simulink model "YawPathControl"  (R2022b)
settings: Solver=VariableStepAuto  StartTime=0.0  StopTime=10  RelTol=1e-3
undefined symbols (not defined in the file): a11, a12, a21, a22, b11, b12, b21, b22, Cf, Cr, Cs, e2, Gn, J, Lf, Lr, m, mu, Q, Vref
libraries: cstblocks x4, slpidlib x1
settings Model: Creator=Santo  LastModifiedBy=brianlesko
settings SolverCC: AlgebraicLoopSolver=TrustRegion
settings DataIOCC: ReturnWorkspaceOutputs=off
settings DebuggingCC: UnconnectedInputMsg=warning  UnconnectedOutputMsg=warning  UnconnectedLineMsg=warning  SFMachineParentedDataDiag=warning  ArithmeticOperatorsInVariantConditions=warning
settings ModelReferenceCC: EnableRefExpFcnMdlSchedulingChecks=on
settings SFSimCC: SimUseLocalCustomCode=off  CustomCodeUndefinedFunction=UseInterfaceOnly
settings RTWCC: RTWUseLocalCustomCode=off

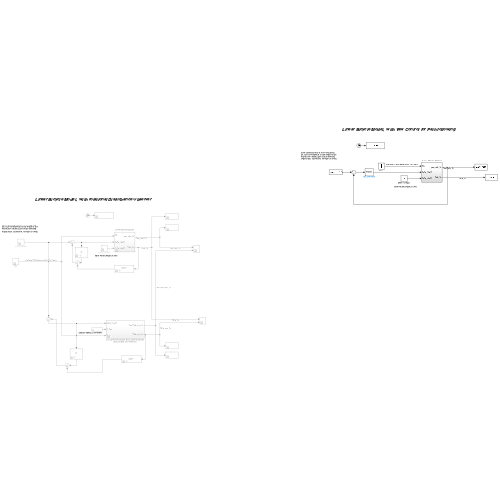
[thumbnail: Simulink's stored preview of the top-level diagram]
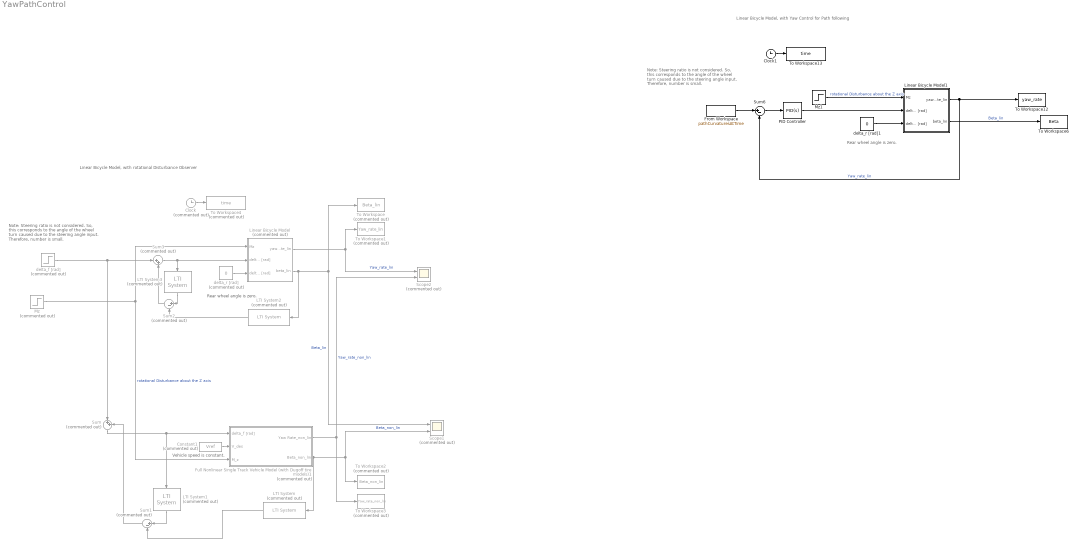
== system YawPathControl ==
  note: Linear Bicycle Model, with rotational Disturbance Observer
  note: Rear wheel angle is zero.
  note: Vehicle speed is constant.
  note: Note: Steering ratio is not considered. So, this corresponds to the angle of the wheel turn caused due to the steering angle input. Therefore, number is small.
  note: Linear Bicycle Model, with Yaw Control for Path following
  note: Rear wheel angle is zero.
  note: Note: Steering ratio is not considered. So, this corresponds to the angle of the wheel turn caused due to the steering angle input. Therefore, number is small.
  Clock : Clock  Commented=on
  Clock1 : Clock
  Constant1 : Constant  Commented=on  Value=Vref
  From Workspace : FromWorkspace  VariableName=pathCurvaturesAtTime
  Full Nonlinear Single Track Vehicle Model (with Dugoff tire models)1 : Subsystem  Commented=on
  LTI System : cstblocks/LTI System  Commented=on  sys=Q/Gn  IC=[]
  LTI System1 : cstblocks/LTI System  Commented=on  sys=Q  IC=[]
  LTI System2 : cstblocks/LTI System  Commented=on  sys=Q/Gn  IC=[]
  LTI System3 : cstblocks/LTI System  Commented=on  sys=Q  IC=[]
  Linear Bicycle Model : Subsystem  Commented=on
  Linear Bicycle Model1 : Subsystem
  Mz : Step  Commented=on  Time=5  After=100  SampleTime=0
  Mz1 : Step  Time=5  After=100  SampleTime=0
  PID Controller : slpidlib/PID Controller  Controller=PID  Form=Parallel  TimeDomain=Continuous-time  UseExternalTs=off  SampleTime=-1  IntegratorMethod=Forward Euler  FilterMethod=Forward Euler  ControllerParametersSource=internal  P=1.20253324681122  I=42.4205335808931  UseKiTs=off  D=0.00143593410548543  N=287.769955007981  UseFilter=on  TunerSelectOption=Transfer Function Based (PID Tuner App)  InitialConditionSource=internal  InitialConditionForIntegrator=0  InitialConditionForFilter=0  DifferentiatorICPrevScaledInput=0  ExternalReset=none  TrackingMode=off  Kt=1  LimitOutput=off  SatLimitsSource=internal  UpperSaturationLimit=inf  LowerSaturationLimit=-inf  LinearizeAsGain=on  AntiWindupMode=none  Kb=1  LimitIntegrator=off  UpperIntegratorSaturationLimit=inf  LowerIntegratorSaturationLimit=-inf  POutMin=[]  POutMax=[]  IOutMin=[]  IOutMax=[]  DOutMin=[]  DOutMax=[]  NOutMin=[]  NOutMax=[]  SumOutMin=[]  SumOutMax=[]  SaturationOutMin=[]  SaturationOutMax=[]  PParamMin=[]  PParamMax=[]  IParamMin=[]  IParamMax=[]  DParamMin=[]  DParamMax=[]  NParamMin=[]  NParamMax=[]  KbParamMin=[]  KbParamMax=[]  KtParamMin=[]  KtParamMax=[]  KbOutMin=[]  KbOutMax=[]  KtOutMin=[]  KtOutMax=[]  IntegratorOutMin=[]  IntegratorOutMax=[]  FilterOutMin=[]  FilterOutMax=[]  SumI1OutMin=[]  SumI1OutMax=[]  SumI2OutMin=[]  SumI2OutMax=[]  SumI3OutMin=[]  SumI3OutMax=[]  SumI4OutMin=[]  SumI4OutMax=[]  SumDOutMin=[]  SumDOutMax=[]  DifferentiatorOutMin=[]  DifferentiatorOutMax=[]  FilterDiffOutCoefMin=[]  FilterDiffOutCoefMax=[]  ReciprocalOutMin=[]  ReciprocalOutMax=[]  SumDenOutMin=[]  SumDenOutMax=[]  SumNumOutMin=[]  SumNumOutMax=[]  DivideOutMin=[]  DivideOutMax=[]  UdiffTsProdOutMin=[]  UdiffTsProdOutMax=[]  NTsProdOutMin=[]  NTsProdOutMax=[]  UintegralTsProdOutMin=[]  UintegralTsProdOutMax=[]  UngainTsProdOutMin=[]  UngainTsProdOutMax=[]  ClampingZeroOutDataTypeStr=Inherit: Inherit via back propagation  ClampingZeroOutMin=[]  ClampingZeroOutMax=[]  FilterDenConstantOutDataTypeStr=Inherit: Inherit via back propagation  FilterDenConstantOutMin=[]  FilterDenConstantOutMax=[]  PCopyOutDataTypeStr=Inherit: Inherit via back propagation  PCopyOutMin=[]  PCopyOutMax=[]  NCopyOutDataTypeStr=Inherit: Inherit via back propagation  NCopyOutMin=[]  NCopyOutMax=[]  IntegratorContinuousStateAttributes=''  IntegratorStateMustResolveToSignalObject=off  IntegratorRTWStateStorageClass=Auto  FilterContinuousStateAttributes=''  FilterStateMustResolveToSignalObject=off  FilterRTWStateStorageClass=Auto  ParallelPVariant=InternalParameters  IdealPVariant=Disabled  IVariant=InternalParameters  DVariant=InternalParameters  IntegratorVariant=Continuous  SatVariant=Disabled  AWVariant=Passthrough  PCopyVariant=Disabled  TRVariant=Disabled  FdbkBlocksVariant=Forward  IdealPFdbkVariant=Disabled  SatFdbkVariant=Disabled  DerivativeFilterVariant=ContFilter  NVariant=InternalParameters  NCopyVariant=Disabled  FilterICVariant=InternalICsFilter  IntegratorICVariant=InternalICs  ExternalResetVariant=Disabled  TRSumVariant=Passthrough  SumFdbkVariant=Disabled  SumVariant=Sum_PID  TsampFilterVariant=InternalTs  TsampNgainVariant=Passthrough  TsampIntegralVariant=Passthrough  ExternalSaturationOutDataTypeStr=Inherit: Same as second input
  Scope1 : Scope  Commented=on  NumInputPorts=2
  Scope2 : Scope  Commented=on  NumInputPorts=2
  Sum : Sum  Commented=on  Inputs=|++
  Sum1 : Sum  Commented=on  Inputs=|+-
  Sum2 : Sum  Commented=on  Inputs=|+-
  Sum3 : Sum  Commented=on  Inputs=|++
  Sum6 : Sum  Inputs=|+-
  To Workspace : ToWorkspace  Commented=on  VariableName=Beta_lin  SampleTime=-1
  To Workspace1 : ToWorkspace  Commented=on  VariableName=Yaw_rate_lin  SampleTime=-1
  To Workspace12 : ToWorkspace  VariableName=yaw_rate  SampleTime=-1
  To Workspace13 : ToWorkspace  VariableName=time  SampleTime=-1
  To Workspace2 : ToWorkspace  Commented=on  VariableName=Beta_non_lin  SampleTime=-1
  To Workspace3 : ToWorkspace  Commented=on  VariableName=Yaw_rate_non_lin  SampleTime=-1
  To Workspace4 : ToWorkspace  Commented=on  VariableName=time  SampleTime=-1
  To Workspace6 : ToWorkspace  VariableName=Beta  SampleTime=-1
  delta_f [rad] : Step  Commented=on  After=5*pi/180  SampleTime=0
  delta_r [rad] : Constant  Commented=on  Value=0
  delta_r [rad]1 : Constant  Value=0
  wires:
  delta_r [rad]/1 -> Linear Bicycle Model/3(delta_r [rad])
  Linear Bicycle Model/1(yaw_rate_lin) -> To Workspace1/1, Scope2/1  "Yaw_rate_lin"
  Linear Bicycle Model/2(beta_lin) -> LTI System2/1, To Workspace/1, Scope1/1  "Beta_lin"
  delta_f [rad]/1 -> Sum3/1, Sum/1
  Full Nonlinear Single Track Vehicle Model (with Dugoff tire models)1/1(Yaw Rate_non_lin) -> To Workspace3/1, Scope2/2  "Yaw_rate_non_lin"
  Mz/1 -> Full Nonlinear Single Track Vehicle Model (with Dugoff tire models)1/3(M_z), Linear Bicycle Model/1(Mz)  "rotational Disturbance about the Z axis"
  Constant1/1 -> Full Nonlinear Single Track Vehicle Model (with Dugoff tire models)1/2("V_des ")
  Full Nonlinear Single Track Vehicle Model (with Dugoff tire models)1/2(Beta_non_lin) -> LTI System/1, To Workspace2/1, Scope1/2  "Beta_non_lin"
  Clock/1 -> To Workspace4/1
  Sum/1 -> Full Nonlinear Single Track Vehicle Model (with Dugoff tire models)1/1(delta_f [rad]), LTI System1/1
  Sum1/1 -> Sum/2
  LTI System1/1 -> Sum1/1
  LTI System/1 -> Sum1/2
  LTI System3/1 -> Sum2/1
  LTI System2/1 -> Sum2/2
  Sum3/1 -> Linear Bicycle Model/2(delta_f [rad]), LTI System3/1
  Sum2/1 -> Sum3/2
  Linear Bicycle Model1/2(beta_lin) -> To Workspace6/1  "Beta_lin"
  Linear Bicycle Model1/1(yaw_rate_lin) -> To Workspace12/1, Sum6/2  "Yaw_rate_lin"
  Mz1/1 -> Linear Bicycle Model1/1(Mz)  "rotational Disturbance about the Z axis"
  Clock1/1 -> To Workspace13/1
  Sum6/1 -> PID Controller/1
  delta_r [rad]1/1 -> Linear Bicycle Model1/3(delta_r [rad])
  PID Controller/1 -> Linear Bicycle Model1/2(delta_f [rad])
  From Workspace/1 -> Sum6/1

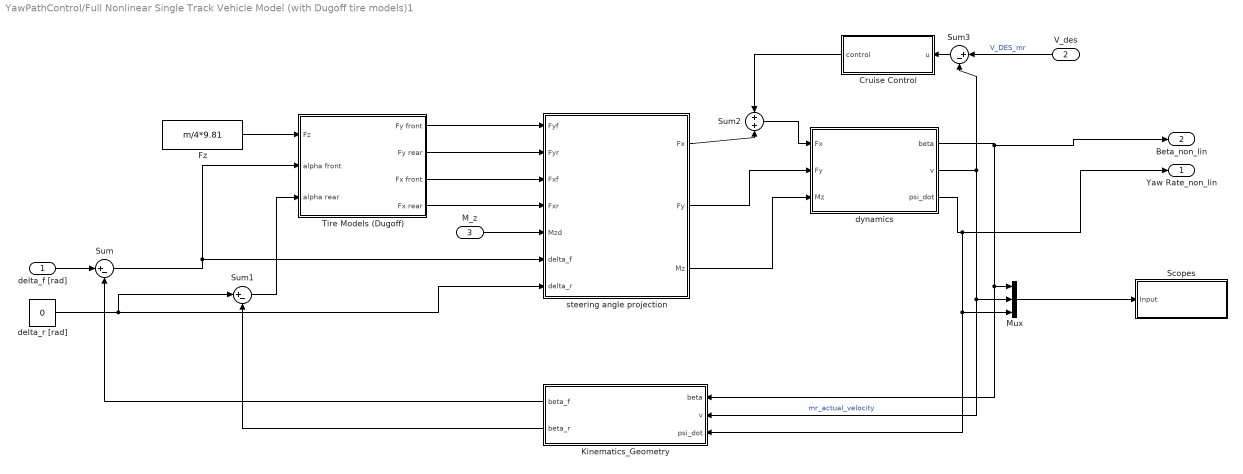
== system YawPathControl/Full Nonlinear Single Track Vehicle Model (with Dugoff tire models)1 ==
  delta_f [rad] : Inport
  "V_des " : Inport  Port=2
  M_z : Inport  Port=3
  Cruise Control : Subsystem
  Fz : Constant  Value=m/4*9.81
  Kinematics_Geometry : Subsystem
  Mux : Mux  Inputs=3
  Scopes : Subsystem
  Sum : Sum  Inputs=|+-  SaturateOnIntegerOverflow=on
  Sum1 : Sum  Inputs=|+-  SaturateOnIntegerOverflow=on
  Sum2 : Sum
  Sum3 : Sum  Inputs=|+-  SaturateOnIntegerOverflow=on
  Tire Models (Dugoff) : Subsystem
  delta_r [rad] : Constant  Value=0
  dynamics : Subsystem
  steering angle projection : Subsystem
  Yaw Rate_non_lin : Outport  VectorParamsAs1DForOutWhenUnconnected=off
  Beta_non_lin : Outport  Port=2  VectorParamsAs1DForOutWhenUnconnected=off
  wires:
  Sum3/1 -> Cruise Control/1(u)
  "V_des "/1 -> Sum3/1  "V_DES_mr"
  steering angle projection/1(Fx) -> Sum2/2
  steering angle projection/2(Fy) -> dynamics/2(Fy)
  steering angle projection/3(Mz) -> dynamics/3(Mz)
  dynamics/2(v) -> Mux/2, Kinematics_Geometry/2(v), Sum3/2  "mr_actual_velocity"
  dynamics/3(psi_dot) -> Yaw Rate_non_lin/1, Mux/3, Kinematics_Geometry/3(psi_dot)
  delta_f [rad]/1 -> Sum/1
  delta_r [rad]/1 -> Sum1/1, steering angle projection/7(delta_r)
  Sum1/1 -> Tire Models (Dugoff)/3(alpha rear)
  Sum/1 -> Tire Models (Dugoff)/2(alpha front), steering angle projection/6(delta_f)
  Mux/1 -> Scopes/1(Input)
  Kinematics_Geometry/1(beta_f) -> Sum/2
  Kinematics_Geometry/2(beta_r) -> Sum1/2
  Fz/1 -> Tire Models (Dugoff)/1(Fz)
  Tire Models (Dugoff)/1(Fy front) -> steering angle projection/1(Fyf)
  Tire Models (Dugoff)/2(Fy rear) -> steering angle projection/2(Fyr)
  Tire Models (Dugoff)/3(Fx front) -> steering angle projection/3(Fxf)
  Tire Models (Dugoff)/4(Fx rear) -> steering angle projection/4(Fxr)
  M_z/1 -> steering angle projection/5(Mzd)
  Cruise Control/1(control) -> Sum2/1
  Sum2/1 -> dynamics/1(Fx)
  dynamics/1(beta) -> Beta_non_lin/1, Kinematics_Geometry/1(beta), Mux/1

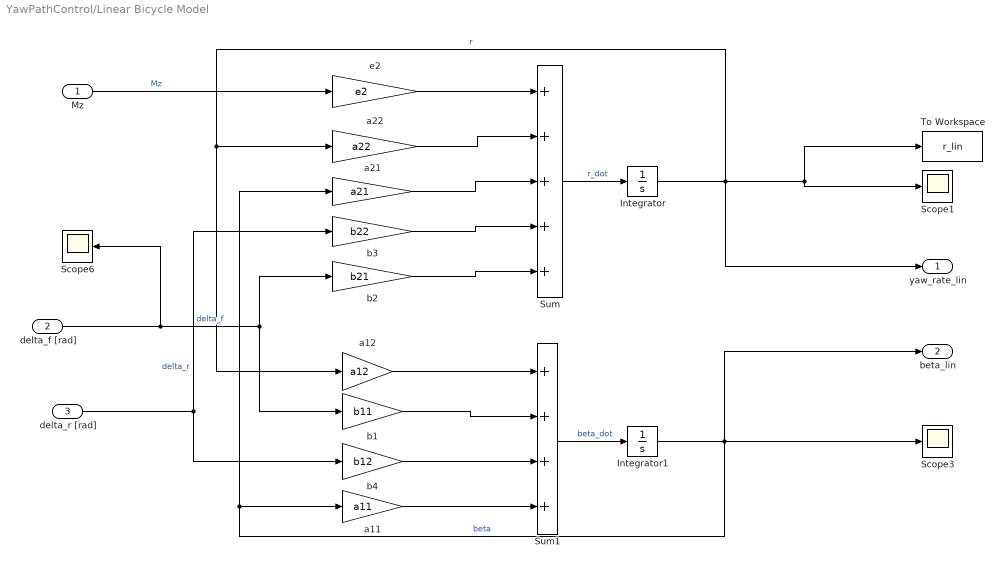
== system YawPathControl/Linear Bicycle Model ==
  Mz : Inport
  delta_f [rad] : Inport  Port=2
  delta_r [rad] : Inport  Port=3
  Integrator : Integrator
  Integrator1 : Integrator
  Scope1 : Scope
  Scope3 : Scope
  Scope6 : Scope
  Sum : Sum  Inputs=+++++
  Sum1 : Sum  Inputs=++++
  To Workspace : ToWorkspace  VariableName=r_lin  SaveFormat=Timeseries  SampleTime=-1
  a11 : Gain  Gain=a11
  a12 : Gain  Gain=a12
  a21 : Gain  Gain=a21
  a22 : Gain  Gain=a22
  b1 : Gain  Gain=b11
  b2 : Gain  Gain=b21
  b3 : Gain  Gain=b22
  b4 : Gain  Gain=b12
  e2 : Gain  Gain=e2
  yaw_rate_lin : Outport  VectorParamsAs1DForOutWhenUnconnected=off
  beta_lin : Outport  Port=2  VectorParamsAs1DForOutWhenUnconnected=off
  wires:
  Sum1/1 -> Integrator1/1  "beta_dot"
  Sum/1 -> Integrator/1  "r_dot"
  a21/1 -> Sum/3
  a11/1 -> Sum1/4
  a12/1 -> Sum1/1
  a22/1 -> Sum/2
  b1/1 -> Sum1/2
  b2/1 -> Sum/5
  delta_f [rad]/1 -> b1/1, b2/1, Scope6/1  "delta_f"
  Integrator1/1 -> beta_lin/1, Scope3/1, a11/1, a21/1  "beta"
  Integrator/1 -> yaw_rate_lin/1, Scope1/1, To Workspace/1, a22/1, a12/1  "r"
  delta_r [rad]/1 -> b3/1, b4/1  "delta_r"
  b3/1 -> Sum/4
  b4/1 -> Sum1/3
  Mz/1 -> e2/1  "Mz"
  e2/1 -> Sum/1

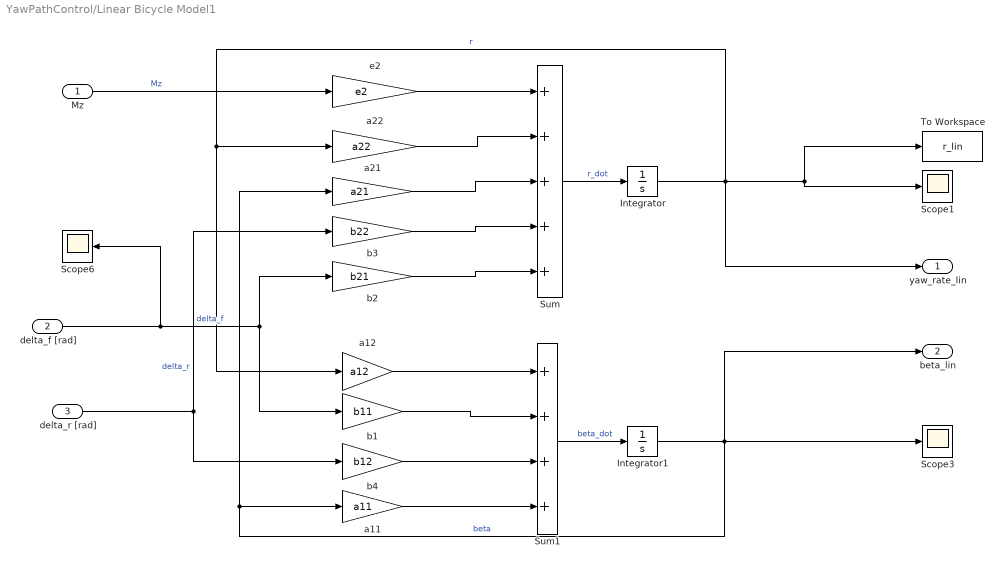
== system YawPathControl/Linear Bicycle Model1 ==
  Mz : Inport
  delta_f [rad] : Inport  Port=2
  delta_r [rad] : Inport  Port=3
  Integrator : Integrator
  Integrator1 : Integrator
  Scope1 : Scope
  Scope3 : Scope
  Scope6 : Scope
  Sum : Sum  Inputs=+++++
  Sum1 : Sum  Inputs=++++
  To Workspace : ToWorkspace  VariableName=r_lin  SaveFormat=Timeseries  SampleTime=-1
  a11 : Gain  Gain=a11
  a12 : Gain  Gain=a12
  a21 : Gain  Gain=a21
  a22 : Gain  Gain=a22
  b1 : Gain  Gain=b11
  b2 : Gain  Gain=b21
  b3 : Gain  Gain=b22
  b4 : Gain  Gain=b12
  e2 : Gain  Gain=e2
  yaw_rate_lin : Outport  VectorParamsAs1DForOutWhenUnconnected=off
  beta_lin : Outport  Port=2  VectorParamsAs1DForOutWhenUnconnected=off
  wires:
  Sum1/1 -> Integrator1/1  "beta_dot"
  Sum/1 -> Integrator/1  "r_dot"
  a21/1 -> Sum/3
  a11/1 -> Sum1/4
  a12/1 -> Sum1/1
  a22/1 -> Sum/2
  b1/1 -> Sum1/2
  b2/1 -> Sum/5
  delta_f [rad]/1 -> b1/1, b2/1, Scope6/1  "delta_f"
  Integrator1/1 -> beta_lin/1, Scope3/1, a11/1, a21/1  "beta"
  Integrator/1 -> yaw_rate_lin/1, Scope1/1, To Workspace/1, a22/1, a12/1  "r"
  delta_r [rad]/1 -> b3/1, b4/1  "delta_r"
  b3/1 -> Sum/4
  b4/1 -> Sum1/3
  Mz/1 -> e2/1  "Mz"
  e2/1 -> Sum/1

== system YawPathControl/Full Nonlinear Single Track Vehicle Model (with Dugoff tire models)1/Cruise Control ==
  u : Inport
  Gain : Gain  Gain=40000  SaturateOnIntegerOverflow=on  OutDataTypeStr=Inherit: Same as input  ParamDataTypeStr=Inherit: Same as input
  Gain1 : Gain  Gain=4000  SaturateOnIntegerOverflow=on  OutDataTypeStr=Inherit: Same as input  ParamDataTypeStr=Inherit: Same as input
  Integrator : Integrator
  Sum : Sum  SaturateOnIntegerOverflow=on
  control : Outport  VectorParamsAs1DForOutWhenUnconnected=off
  wires:
  u/1 -> Gain/1, Integrator/1
  Integrator/1 -> Gain1/1
  Gain1/1 -> Sum/2
  Gain/1 -> Sum/1
  Sum/1 -> control/1

== system YawPathControl/Full Nonlinear Single Track Vehicle Model (with Dugoff tire models)1/Kinematics_Geometry ==
  beta : Inport
  v : Inport  Port=2
  psi_dot : Inport  Port=3
  Mux : Mux  Inputs=3
  beta_f Calc : Fcn  Expr=atan( tan(u(1)) + u(3)*Lf/(u(2)*cos(u(1))) )
  beta_r Calc : Fcn  Expr=atan( tan(u(1)) - u(3)*Lr/(u(2)*cos(u(1))) )
  beta_f : Outport  VectorParamsAs1DForOutWhenUnconnected=off
  beta_r : Outport  Port=2  VectorParamsAs1DForOutWhenUnconnected=off
  wires:
  beta/1 -> Mux/1
  v/1 -> Mux/2
  psi_dot/1 -> Mux/3
  Mux/1 -> beta_f Calc/1, beta_r Calc/1
  beta_r Calc/1 -> beta_r/1
  beta_f Calc/1 -> beta_f/1

== system YawPathControl/Full Nonlinear Single Track Vehicle Model (with Dugoff tire models)1/Scopes ==
  Input : Inport
  Demux : Demux  Outputs=3
      settings: DisplayOption=none
  Distance Traveled : Subsystem
  beta : Scope
  speed : Scope
  yaw Calc : Integrator
  yaw angle : Scope
  yaw rate : Scope
  wires:
  Input/1 -> Demux/1
  Demux/1 -> beta/1, Distance Traveled/2(beta)
  Demux/2 -> speed/1, Distance Traveled/1(V)
  Demux/3 -> yaw rate/1, yaw Calc/1
  yaw Calc/1 -> yaw angle/1, Distance Traveled/3(psi)

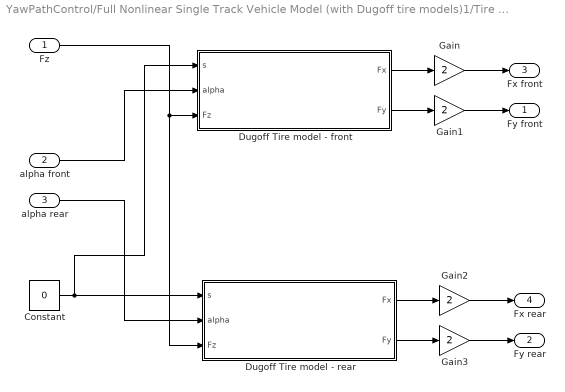
== system YawPathControl/Full Nonlinear Single Track Vehicle Model (with Dugoff tire models)1/Tire Models (Dugoff) ==
  Fz : Inport
  alpha front : Inport  Port=2
  alpha rear : Inport  Port=3
  Constant : Constant  Value=0
  Dugoff Tire model - front : Subsystem
  Dugoff Tire model - rear : Subsystem
  Gain{,1..3} (4 alike) : Gain  Gain=2
  Fy front : Outport  VectorParamsAs1DForOutWhenUnconnected=off
  Fy rear : Outport  Port=2  VectorParamsAs1DForOutWhenUnconnected=off
  Fx front : Outport  Port=3  VectorParamsAs1DForOutWhenUnconnected=off
  Fx rear : Outport  Port=4  VectorParamsAs1DForOutWhenUnconnected=off
  wires:
  alpha rear/1 -> Dugoff Tire model - rear/2(alpha)
  alpha front/1 -> Dugoff Tire model - front/2(alpha)
  Fz/1 -> Dugoff Tire model - front/3(Fz), Dugoff Tire model - rear/3(Fz)
  Constant/1 -> Dugoff Tire model - front/1(s), Dugoff Tire model - rear/1(s)
  Dugoff Tire model - rear/2(Fy) -> Gain3/1
  Dugoff Tire model - rear/1(Fx) -> Gain2/1
  Dugoff Tire model - front/2(Fy) -> Gain1/1
  Dugoff Tire model - front/1(Fx) -> Gain/1
  Gain/1 -> Fx front/1
  Gain1/1 -> Fy front/1
  Gain2/1 -> Fx rear/1
  Gain3/1 -> Fy rear/1

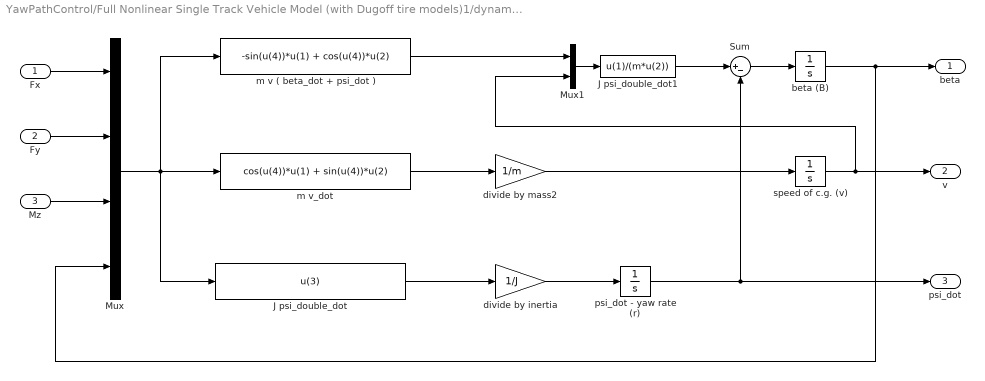
== system YawPathControl/Full Nonlinear Single Track Vehicle Model (with Dugoff tire models)1/dynamics ==
  Fx : Inport
  Fy : Inport  Port=2
  Mz : Inport  Port=3
  J psi_double_dot : Fcn  Expr=u(3)
  J psi_double_dot1 : Fcn  Expr=u(1)/(m*u(2))
  Mux : Mux
  Mux1 : Mux  Inputs=2
  Sum : Sum  Inputs=|+-  SaturateOnIntegerOverflow=on
  beta (B) : Integrator
  divide by inertia : Gain  Gain=1/J  SaturateOnIntegerOverflow=on  OutDataTypeStr=Inherit: Same as input  ParamDataTypeStr=Inherit: Same as input
  divide by mass2 : Gain  Gain=1/m  SaturateOnIntegerOverflow=on  OutDataTypeStr=Inherit: Same as input  ParamDataTypeStr=Inherit: Same as input
  m v ( beta_dot + psi_dot ) : Fcn  Expr=-sin(u(4))*u(1) + cos(u(4))*u(2)
  m v_dot : Fcn  Expr=cos(u(4))*u(1) + sin(u(4))*u(2)
  psi_dot - yaw rate (r) : Integrator
  speed of c.g. (v) : Integrator  InitialCondition=Vref
  beta : Outport  VectorParamsAs1DForOutWhenUnconnected=off
  v : Outport  Port=2  VectorParamsAs1DForOutWhenUnconnected=off
  psi_dot : Outport  Port=3  VectorParamsAs1DForOutWhenUnconnected=off
  wires:
  Fx/1 -> Mux/1
  Fy/1 -> Mux/2
  Mz/1 -> Mux/3
  Mux/1 -> m v ( beta_dot + psi_dot )/1, m v_dot/1, J psi_double_dot/1
  divide by inertia/1 -> psi_dot - yaw rate (r)/1
  Sum/1 -> beta (B)/1
  psi_dot - yaw rate (r)/1 -> Sum/2, psi_dot/1
  divide by mass2/1 -> speed of c.g. (v)/1
  speed of c.g. (v)/1 -> v/1, Mux1/2
  beta (B)/1 -> beta/1, Mux/4
  m v ( beta_dot + psi_dot )/1 -> Mux1/1
  m v_dot/1 -> divide by mass2/1
  J psi_double_dot/1 -> divide by inertia/1
  Mux1/1 -> J psi_double_dot1/1
  J psi_double_dot1/1 -> Sum/1

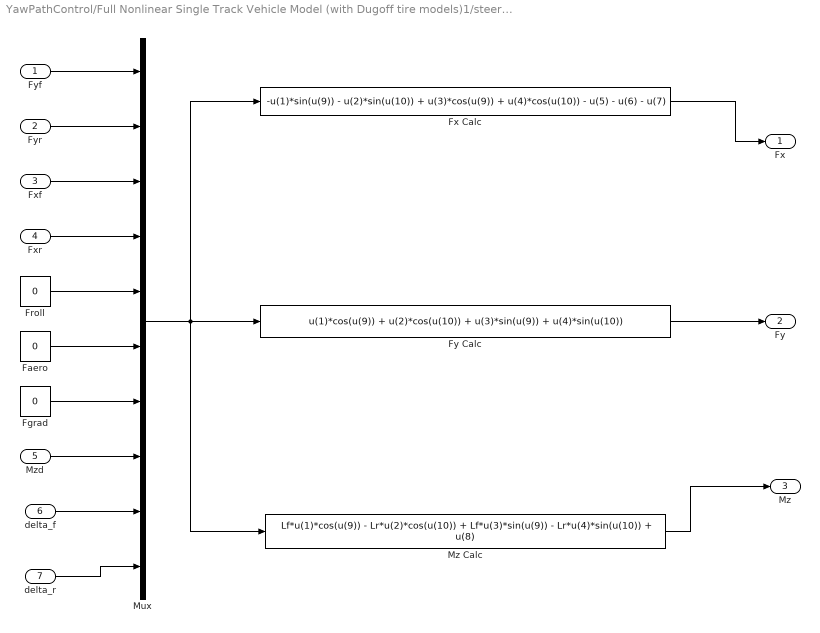
== system YawPathControl/Full Nonlinear Single Track Vehicle Model (with Dugoff tire models)1/steering angle projection ==
  Fyf : Inport
  Fyr : Inport  Port=2
  Fxf : Inport  Port=3
  Fxr : Inport  Port=4
  Mzd : Inport  Port=5
  delta_f : Inport  Port=6
  delta_r : Inport  Port=7
  Faero : Constant  Value=0
  Fgrad : Constant  Value=0
  Froll : Constant  Value=0
  Fx Calc : Fcn  Expr=-u(1)*sin(u(9)) - u(2)*sin(u(10)) + u(3)*cos(u(9)) + u(4)*cos(u(10)) - u(5) - u(6) - u(7)
  Fy Calc : Fcn  Expr=u(1)*cos(u(9)) + u(2)*cos(u(10)) + u(3)*sin(u(9)) + u(4)*sin(u(10))
  Mux : Mux  Inputs=10
  Mz Calc : Fcn  Expr=Lf*u(1)*cos(u(9)) - Lr*u(2)*cos(u(10)) + Lf*u(3)*sin(u(9)) - Lr*u(4)*sin(u(10)) + u(8)
  Fx : Outport  VectorParamsAs1DForOutWhenUnconnected=off
  Fy : Outport  Port=2  VectorParamsAs1DForOutWhenUnconnected=off
  Mz : Outport  Port=3  VectorParamsAs1DForOutWhenUnconnected=off
  wires:
  Fyf/1 -> Mux/1
  Fyr/1 -> Mux/2
  Fxf/1 -> Mux/3
  Fxr/1 -> Mux/4
  Froll/1 -> Mux/5
  Faero/1 -> Mux/6
  Fgrad/1 -> Mux/7
  Mzd/1 -> Mux/8
  delta_f/1 -> Mux/9
  delta_r/1 -> Mux/10
  Fx Calc/1 -> Fx/1
  Mux/1 -> Fx Calc/1, Fy Calc/1, Mz Calc/1
  Fy Calc/1 -> Fy/1
  Mz Calc/1 -> Mz/1

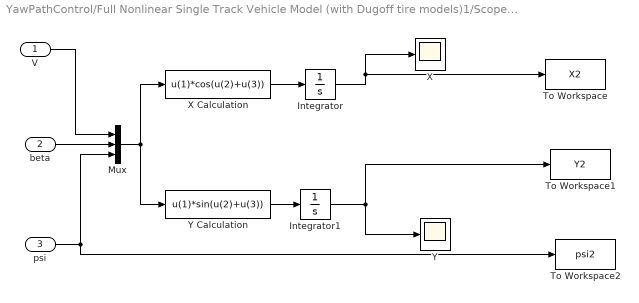
== system YawPathControl/Full Nonlinear Single Track Vehicle Model (with Dugoff tire models)1/Scopes/Distance Traveled ==
  V : Inport
  beta : Inport  Port=2
  psi : Inport  Port=3
  Integrator : Integrator
  Integrator1 : Integrator
  Mux : Mux  Inputs=3
  To Workspace : ToWorkspace  VariableName=X2  SampleTime=-1
  To Workspace1 : ToWorkspace  VariableName=Y2  SampleTime=-1
  To Workspace2 : ToWorkspace  VariableName=psi2  SampleTime=-1
  X : Scope
  X Calculation : Fcn  Expr=u(1)*cos(u(2)+u(3))
  Y : Scope
  Y Calculation : Fcn  Expr=u(1)*sin(u(2)+u(3))
  wires:
  Y Calculation/1 -> Integrator1/1
  X Calculation/1 -> Integrator/1
  Mux/1 -> Y Calculation/1, X Calculation/1
  psi/1 -> Mux/3, To Workspace2/1
  beta/1 -> Mux/2
  V/1 -> Mux/1
  Integrator/1 -> X/1, To Workspace/1
  Integrator1/1 -> Y/1, To Workspace1/1

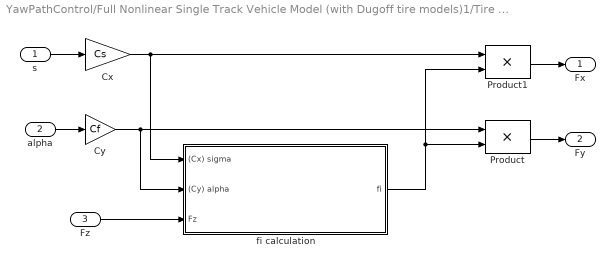
== system YawPathControl/Full Nonlinear Single Track Vehicle Model (with Dugoff tire models)1/Tire Models (Dugoff)/Dugoff Tire model - front ==
  s : Inport
  alpha : Inport  Port=2
  Fz : Inport  Port=3
  Cx : Gain  Gain=Cs  SaturateOnIntegerOverflow=on  OutDataTypeStr=Inherit: Same as input  ParamDataTypeStr=Inherit: Same as input
  Cy : Gain  Gain=Cf  SaturateOnIntegerOverflow=on  OutDataTypeStr=Inherit: Same as input  ParamDataTypeStr=Inherit: Same as input
  Product : Product  SaturateOnIntegerOverflow=on  OutDataTypeStr=Inherit: Same as first input
  Product1 : Product  SaturateOnIntegerOverflow=on  OutDataTypeStr=Inherit: Same as first input
  fi calculation : Subsystem
  Fx : Outport  VectorParamsAs1DForOutWhenUnconnected=off
  Fy : Outport  Port=2  VectorParamsAs1DForOutWhenUnconnected=off
  wires:
  s/1 -> Cx/1
  alpha/1 -> Cy/1
  Cy/1 -> Product/1, fi calculation/2((Cy) alpha)
  Cx/1 -> Product1/1, fi calculation/1((Cx) sigma)
  Product/1 -> Fy/1
  Product1/1 -> Fx/1
  fi calculation/1(fi) -> Product/2, Product1/2
  Fz/1 -> fi calculation/3(Fz)

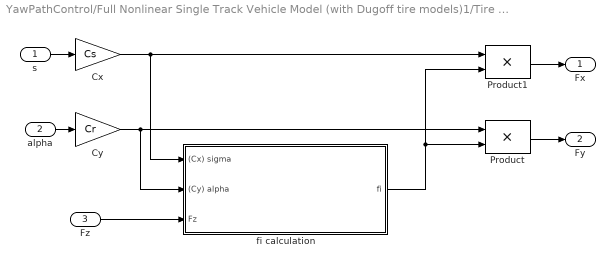
== system YawPathControl/Full Nonlinear Single Track Vehicle Model (with Dugoff tire models)1/Tire Models (Dugoff)/Dugoff Tire model - rear ==
  s : Inport
  alpha : Inport  Port=2
  Fz : Inport  Port=3
  Cx : Gain  Gain=Cs  SaturateOnIntegerOverflow=on  OutDataTypeStr=Inherit: Same as input  ParamDataTypeStr=Inherit: Same as input
  Cy : Gain  Gain=Cr  SaturateOnIntegerOverflow=on  OutDataTypeStr=Inherit: Same as input  ParamDataTypeStr=Inherit: Same as input
  Product : Product  SaturateOnIntegerOverflow=on  OutDataTypeStr=Inherit: Same as first input
  Product1 : Product  SaturateOnIntegerOverflow=on  OutDataTypeStr=Inherit: Same as first input
  fi calculation : Subsystem
  Fx : Outport  VectorParamsAs1DForOutWhenUnconnected=off
  Fy : Outport  Port=2  VectorParamsAs1DForOutWhenUnconnected=off
  wires:
  Fz/1 -> fi calculation/3(Fz)
  fi calculation/1(fi) -> Product1/2, Product/2
  Product1/1 -> Fx/1
  Product/1 -> Fy/1
  Cx/1 -> fi calculation/1((Cx) sigma), Product1/1
  Cy/1 -> fi calculation/2((Cy) alpha), Product/1
  alpha/1 -> Cy/1
  s/1 -> Cx/1

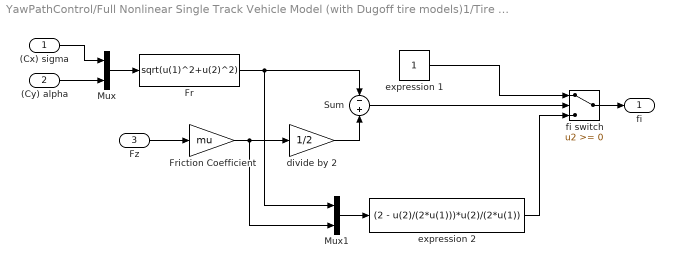
== system YawPathControl/Full Nonlinear Single Track Vehicle Model (with Dugoff tire models)1/Tire Models (Dugoff)/Dugoff Tire model - front/fi calculation ==
  (Cx) sigma : Inport
  (Cy) alpha : Inport  Port=2
  Fz : Inport  Port=3
  Fr : Fcn  Expr=sqrt(u(1)^2+u(2)^2)
  Friction Coefficient : Gain  Gain=mu  SaturateOnIntegerOverflow=on  OutDataTypeStr=Inherit: Same as input  ParamDataTypeStr=Inherit: Same as input
  Mux : Mux  Inputs=2
  Mux1 : Mux  Inputs=2
  Sum : Sum  Inputs=-+  SaturateOnIntegerOverflow=on
  divide by 2 : Gain  Gain=1/2  SaturateOnIntegerOverflow=on  OutDataTypeStr=Inherit: Same as input  ParamDataTypeStr=Inherit: Same as input
  expression 1 : Constant
  expression 2 : Fcn  Expr=(2 - u(2)/(2*u(1)))*u(2)/(2*u(1))
  fi switch : Switch  InputSameDT=off
  fi : Outport  VectorParamsAs1DForOutWhenUnconnected=off
  wires:
  Mux/1 -> Fr/1
  Fz/1 -> Friction Coefficient/1
  Sum/1 -> fi switch/2
  Fr/1 -> Sum/1, Mux1/1
  Friction Coefficient/1 -> Mux1/2, divide by 2/1
  expression 1/1 -> fi switch/1
  Mux1/1 -> expression 2/1
  expression 2/1 -> fi switch/3
  divide by 2/1 -> Sum/2
  (Cx) sigma/1 -> Mux/1
  (Cy) alpha/1 -> Mux/2
  fi switch/1 -> fi/1

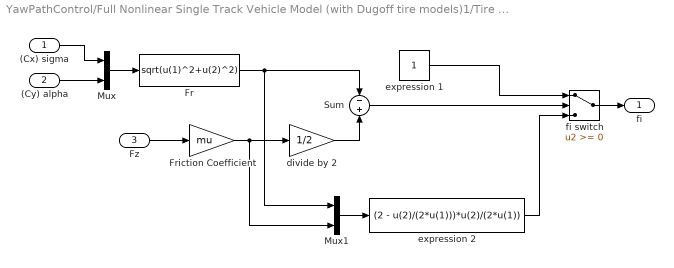
== system YawPathControl/Full Nonlinear Single Track Vehicle Model (with Dugoff tire models)1/Tire Models (Dugoff)/Dugoff Tire model - rear/fi calculation ==
  (Cx) sigma : Inport
  (Cy) alpha : Inport  Port=2
  Fz : Inport  Port=3
  Fr : Fcn  Expr=sqrt(u(1)^2+u(2)^2)
  Friction Coefficient : Gain  Gain=mu  SaturateOnIntegerOverflow=on  OutDataTypeStr=Inherit: Same as input  ParamDataTypeStr=Inherit: Same as input
  Mux : Mux  Inputs=2
  Mux1 : Mux  Inputs=2
  Sum : Sum  Inputs=-+  SaturateOnIntegerOverflow=on
  divide by 2 : Gain  Gain=1/2  SaturateOnIntegerOverflow=on  OutDataTypeStr=Inherit: Same as input  ParamDataTypeStr=Inherit: Same as input
  expression 1 : Constant
  expression 2 : Fcn  Expr=(2 - u(2)/(2*u(1)))*u(2)/(2*u(1))
  fi switch : Switch  InputSameDT=off
  fi : Outport  VectorParamsAs1DForOutWhenUnconnected=off
  wires:
  fi switch/1 -> fi/1
  (Cy) alpha/1 -> Mux/2
  (Cx) sigma/1 -> Mux/1
  divide by 2/1 -> Sum/2
  expression 2/1 -> fi switch/3
  Mux1/1 -> expression 2/1
  expression 1/1 -> fi switch/1
  Friction Coefficient/1 -> divide by 2/1, Mux1/2
  Fr/1 -> Mux1/1, Sum/1
  Sum/1 -> fi switch/2
  Fz/1 -> Friction Coefficient/1
  Mux/1 -> Fr/1
